simulink model "Aeropendulum"  (R2018b)
settings: Solver=VariableStepAuto  StartTime=0.0  StopTime=5  FixedStep=1e-3  MaxStep=1e-3  RelTol=1e-3
InitFcn:
  | mm = (0.008+0.0004+0.0034+2*0.0024);
  | mh = 0.007;
  | r = 0.012;
  | L = 0.285;
  | J = (mh*L^2)/3 + (2*mm*r^2)/5 + mm*(L+r)^2;
  | 
  | 
  | % where: mm = mass of the motor-propeller assembly
  | %            mh  = mass of the rod
  | 
  | coef = 0.0074;
  | 
  | A = -3.8099e-3;
  | B = 39.1002e-3;
  | C =  3.1245e-3;
  | D =  0;
  | 
  | fcpb = 2000;
libraries: simulink x1, vrlib x1, powerlib x1
settings Model: Creator=user  LastModifiedBy=user
settings CodeAppCC: StateflowObjectComments=on

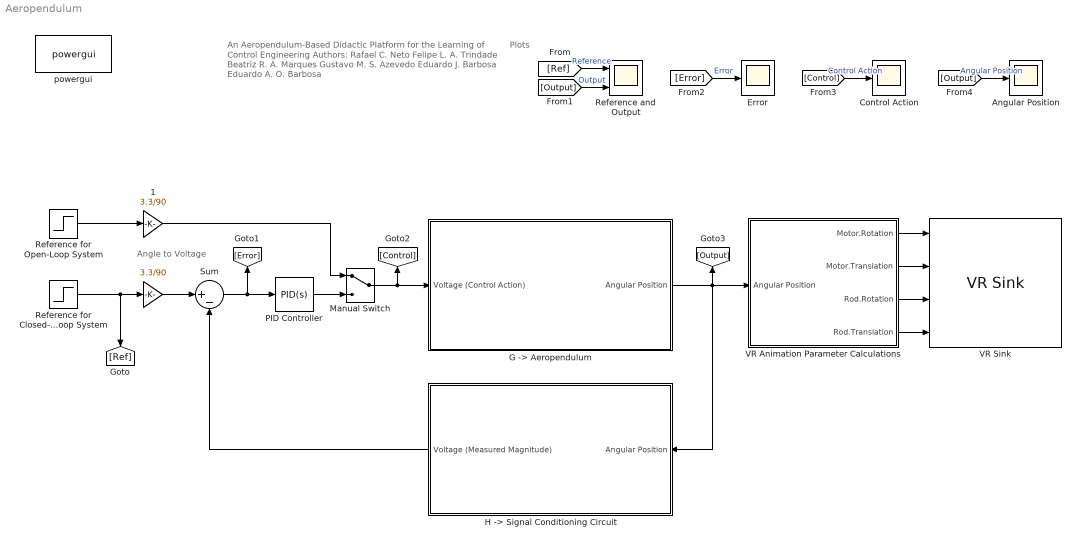
== system Aeropendulum ==
  note: Plots
  note: Angle to
      | Voltage
  note: An Aeropendulum-Based Didactic Platform
      | for the Learning of Control Engineering
      |
      | Authors: Rafael C. Neto
      | Felipe L. A. Trindade
      | Beatriz R. A. Marques
      | Gustavo M. S. Azevedo
      | Eduardo J. Barbosa
      | Eduardo A. O. Barbosa
  " " : Gain  Gain=3.3/90
  " 1" : Gain  Gain=3.3/90
  Angular Position : Scope
  Control Action : Scope
  Error : Scope
  "G -> Aeropendulum" : Subsystem  InitFcn=|
      | mm = (8+0.4+3.4+2*2.4)/1000  ; % motor + helice + parafusos + acrilico
      | mh = 0.007;
      | r = 0.03;
      | l = 0.25;
      | J = (mh*l^2/2) + (2*mm*r^2)/5 + mm*l^2;
  "H -> Signal Conditioning Circuit" : Subsystem
  Manual Switch : ManualSwitch
  PID Controller : simulink/Continuous/PID Controller  Controller=PID  Form=Parallel  TimeDomain=Continuous-time  SampleTime=-1  IntegratorMethod=Forward Euler  FilterMethod=Forward Euler  ControllerParametersSource=internal  P=0.095  I=0.95  D=0  UseFilter=on  N=100  TunerSelectOption=Transfer Function Based (PID Tuner App)  InitialConditionSource=internal  InitialConditionForIntegrator=0  InitialConditionForFilter=0  DifferentiatorICPrevScaledInput=0  ExternalReset=none  TrackingMode=off  Kt=1  LimitOutput=off  UpperSaturationLimit=inf  LowerSaturationLimit=-inf  LinearizeAsGain=on  AntiWindupMode=none  Kb=1  POutMin=[]  POutMax=[]  IOutMin=[]  IOutMax=[]  DOutMin=[]  DOutMax=[]  NOutMin=[]  NOutMax=[]  SumOutMin=[]  SumOutMax=[]  SaturationOutMin=[]  SaturationOutMax=[]  PParamMin=[]  PParamMax=[]  IParamMin=[]  IParamMax=[]  DParamMin=[]  DParamMax=[]  NParamMin=[]  NParamMax=[]  KbParamMin=[]  KbParamMax=[]  KtParamMin=[]  KtParamMax=[]  KbOutMin=[]  KbOutMax=[]  KtOutMin=[]  KtOutMax=[]  IntegratorOutMin=[]  IntegratorOutMax=[]  FilterOutMin=[]  FilterOutMax=[]  SumI1OutMin=[]  SumI1OutMax=[]  SumI2OutMin=[]  SumI2OutMax=[]  SumI3OutMin=[]  SumI3OutMax=[]  SumI4OutMin=[]  SumI4OutMax=[]  SumDOutMin=[]  SumDOutMax=[]  DifferentiatorOutMin=[]  DifferentiatorOutMax=[]  FilterDiffOutCoefMin=[]  FilterDiffOutCoefMax=[]  ReciprocalOutMin=[]  ReciprocalOutMax=[]  SumDenOutMin=[]  SumDenOutMax=[]  SumNumOutMin=[]  SumNumOutMax=[]  DivideOutMin=[]  DivideOutMax=[]  IntegratorContinuousStateAttributes=''  IntegratorStateMustResolveToSignalObject=off  IntegratorRTWStateStorageClass=Auto  FilterContinuousStateAttributes=''  FilterStateMustResolveToSignalObject=off  FilterRTWStateStorageClass=Auto  ParallelPVariant=InternalParameters  IdealPVariant=Disabled  IVariant=InternalParameters  DVariant=InternalParameters  IntegratorVariant=Continuous  SatVariant=Disabled  AWVariant=Passthrough  PCopyVariant=Disabled  TRVariant=Disabled  FdbkBlocksVariant=Forward  IdealPFdbkVariant=Disabled  SatFdbkVariant=Disabled  DerivativeFilterVariant=ContFilter  NVariant=InternalParameters  NCopyVariant=Disabled  FilterICVariant=InternalICsFilter  IntegratorICVariant=InternalICs  ExternalResetVariant=Disabled  TRSumVariant=Passthrough  SumFdbkVariant=Disabled  SumVariant=Sum_PID
  Reference and Output : Scope  NumInputPorts=2
  Reference for Closed-Loop System : Step  After=55  SampleTime=0
  Reference for Open-Loop System : Step  After=55  SampleTime=0
  Sum : Sum  Inputs=|+-
  VR Animation Parameter Calculations : Subsystem
  VR Sink : vrlib/VR Sink  InstantiateOnLoad=on  SampleTime=0.01  ViewEnable=on  RemoteChange=off  RemoteView=off  FieldsWritten=Motor.rotation.4.1.1.double#Motor.translation.3.1.1.double#Haste.rotation.4.1.1.double#Haste.translation.3.1.1.double  WorldFileName=VRML_Aeropendulum.WRL  AutoView=off  VideoDimensions=[]  AllowVariableSize=off
      settings: SourceProductName=Simulink
  powergui : powerlib/powergui  Priority=1  SimulationMode=Discrete  SampleTime=1e-3  frequency=60  Iterations=50  frequencyindice=0  Pbase=100e6  ErrMax=1e-4  UnitsV=kV  UnitsW=MW  buscounter=0  FunctionMessages=off  echomessages=off  EnableUseOfTLC=off  CurrentSourceSwitches=off  DisableSnubberDevices=off  DisableRonSwitches=off  DisableVfSwitches=off  DisplayEquations=off  SolverType=Tustin/Backward Euler (TBE)  Interpol=off  ExternalGateDelay=off  methode=off  Ts=100  x0status=blocks  SPID=off  SwTol=0  HookPort=off  RestoreLinks=warning  ResistiveCurrentMeasurement=off  Frange=[0:2:500]  Ylog=off  Xlog=on  ShowGrid=off  save=off  variable=ZData  structure=0  ZoomFFT=off  StartTime=0.0  cycles=1  DisplayStyle=1  fundamental=60  FreqAxis=off  MaxFrequency=1000  frequencyindicesteady=1  RmsSteady=1  display=off
  wires:
  "G -> Aeropendulum"/1(Angular Position) -> "H -> Signal Conditioning Circuit"/1(Angular Position), VR Animation Parameter Calculations/1(Angular Position), [Output]
  "H -> Signal Conditioning Circuit"/1(Voltage (Measured Magnitude)) -> Sum/2
  Reference for Closed-Loop System/1 -> " "/1, [Ref]
  Sum/1 -> PID Controller/1, [Error]
  VR Animation Parameter Calculations/1(Motor.Rotation) -> VR Sink/1
  VR Animation Parameter Calculations/2(Motor.Translation) -> VR Sink/2
  VR Animation Parameter Calculations/3(Rod.Rotation) -> VR Sink/3
  VR Animation Parameter Calculations/4(Rod.Translation) -> VR Sink/4
  Manual Switch/1 -> "G -> Aeropendulum"/1(Voltage (Control Action)), [Control]
  Reference for Open-Loop System/1 -> " 1"/1
  PID Controller/1 -> Manual Switch/2
  " "/1 -> Sum/1
  [Ref] -> Reference and Output/1  "Reference"
  [Output] -> Reference and Output/2  "Output"
  [Error] -> Error/1  "Error"
  [Control] -> Control Action/1  "Control Action"
  [Output] -> Angular Position/1  "Angular Position"
  " 1"/1 -> Manual Switch/1

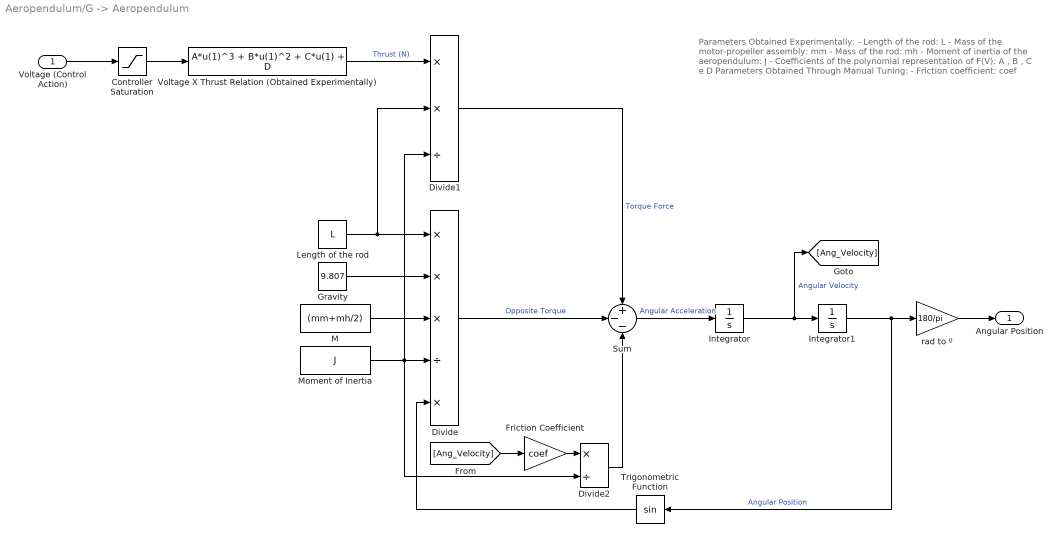
== system Aeropendulum/G -> Aeropendulum ==
  note: Parameters Obtained Experimentally:
      | - Length of the rod: L
      | - Mass of the motor-propeller assembly: mm
      | - Mass of the rod: mh
      | - Moment of inertia of the aeropendulum: J
      | - Coefficients of the polynomial
      | representation of F(V): A , B , C e D
      |
      | Parameters Obtained Through Manual Tuning:
      | - Friction coefficient: coef
  Voltage (Control Action) : Inport
  " Friction Coefficient" : Gain  Gain=coef
  Controller Saturation : Saturate  UpperLimit=3.7  LowerLimit=0
  Divide : Product  Inputs=***/*
  Divide1 : Product  Inputs=**/
  Divide2 : Product  Inputs=*/
  Gravity : Constant  Value=9.807
  Integrator : Integrator
  Integrator1 : Integrator
  Length of the rod : Constant  Value=L
  M : Constant  Value=(mm+mh/2)
  Moment of Inertia : Constant  Value=J
  Sum : Sum  Inputs=+--
  Trigonometric Function : Trigonometry
  Voltage X Thrust Relation (Obtained Experimentally) : Fcn  Expr=A*u(1)^3 + B*u(1)^2 + C*u(1) + D
  rad to º : Gain  Gain=180/pi
  Angular Position : Outport
  wires:
  Trigonometric Function/1 -> Divide/5
  Length of the rod/1 -> Divide1/2, Divide/1
  Moment of Inertia/1 -> Divide2/2, Divide1/3, Divide/4
  M/1 -> Divide/3
  Voltage (Control Action)/1 -> Controller Saturation/1
  Voltage X Thrust Relation (Obtained Experimentally)/1 -> Divide1/1  "Thrust (N)"
  Gravity/1 -> Divide/2
  Integrator/1 -> [Ang_Velocity], Integrator1/1  "Angular Velocity"
  Sum/1 -> Integrator/1  "Angular Acceleration"
  Integrator1/1 -> rad to º/1, Trigonometric Function/1  "Angular Position"
  Divide/1 -> Sum/2  "Opposite Torque"
  rad to º/1 -> Angular Position/1
  Divide1/1 -> Sum/1  "Torque Force"
  Controller Saturation/1 -> Voltage X Thrust Relation (Obtained Experimentally)/1
  [Ang_Velocity] -> " Friction Coefficient"/1
  " Friction Coefficient"/1 -> Divide2/1
  Divide2/1 -> Sum/3

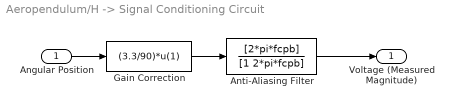
== system Aeropendulum/H -> Signal Conditioning Circuit ==
  Angular Position : Inport
  Anti-Aliasing Filter : TransferFcn  Numerator=[2*pi*fcpb]  Denominator=[1 2*pi*fcpb]
  Gain Correction : Fcn  Expr=(3.3/90)*u(1)
  Voltage (Measured Magnitude) : Outport
  wires:
  Gain Correction/1 -> Anti-Aliasing Filter/1
  Angular Position/1 -> Gain Correction/1
  Anti-Aliasing Filter/1 -> Voltage (Measured Magnitude)/1

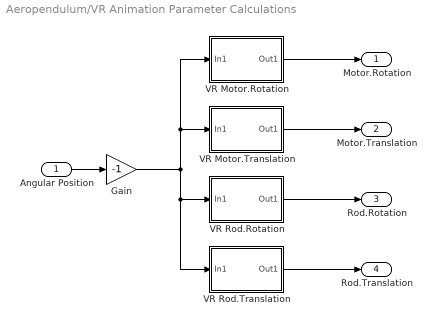
== system Aeropendulum/VR Animation Parameter Calculations ==
  Angular Position : Inport
  Gain : Gain  Gain=-1
  VR Motor.Rotation : Subsystem
  VR Motor.Translation : Subsystem
  VR Rod.Rotation : Subsystem
  VR Rod.Translation : Subsystem
  Motor.Rotation : Outport
  Motor.Translation : Outport  Port=2
  Rod.Rotation : Outport  Port=3
  Rod.Translation : Outport  Port=4
  wires:
  VR Rod.Translation/1(Out1) -> Rod.Translation/1
  Angular Position/1 -> Gain/1
  VR Rod.Rotation/1(Out1) -> Rod.Rotation/1
  VR Motor.Translation/1(Out1) -> Motor.Translation/1
  VR Motor.Rotation/1(Out1) -> Motor.Rotation/1
  Gain/1 -> VR Motor.Rotation/1(In1), VR Motor.Translation/1(In1), VR Rod.Translation/1(In1), VR Rod.Rotation/1(In1)

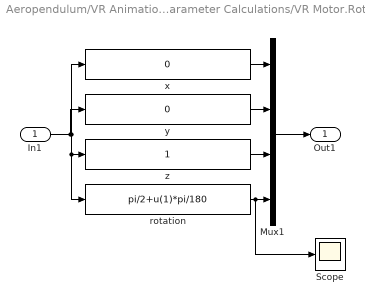
== system Aeropendulum/VR Animation Parameter Calculations/VR Motor.Rotation ==
  In1 : Inport
  Mux1 : Mux
  Scope : Scope
  rotation : Fcn  Expr=pi/2+u(1)*pi/180
  x : Fcn  Expr=0
  y : Fcn  Expr=0
  z : Fcn  Expr=1
  Out1 : Outport
  wires:
  Mux1/1 -> Out1/1
  In1/1 -> y/1, z/1, rotation/1, x/1
  y/1 -> Mux1/2
  x/1 -> Mux1/1
  rotation/1 -> Scope/1, Mux1/4
  z/1 -> Mux1/3

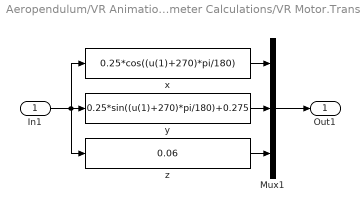
== system Aeropendulum/VR Animation Parameter Calculations/VR Motor.Translation ==
  In1 : Inport
  Mux1 : Mux  Inputs=3
  x : Fcn  Expr=0.25*cos((u(1)+270)*pi/180)
  y : Fcn  Expr=0.25*sin((u(1)+270)*pi/180)+0.275
  z : Fcn  Expr=0.06
  Out1 : Outport
  wires:
  x/1 -> Mux1/1
  y/1 -> Mux1/2
  In1/1 -> x/1, z/1, y/1
  z/1 -> Mux1/3
  Mux1/1 -> Out1/1

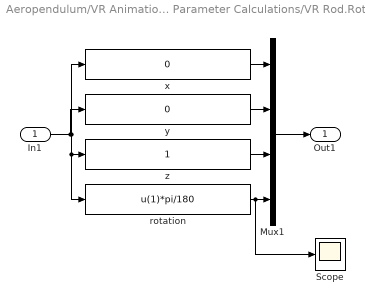
== system Aeropendulum/VR Animation Parameter Calculations/VR Rod.Rotation ==
  In1 : Inport
  Mux1 : Mux
  Scope : Scope
  rotation : Fcn  Expr=u(1)*pi/180
  x : Fcn  Expr=0
  y : Fcn  Expr=0
  z : Fcn  Expr=1
  Out1 : Outport
  wires:
  Mux1/1 -> Out1/1
  In1/1 -> y/1, z/1, rotation/1, x/1
  y/1 -> Mux1/2
  x/1 -> Mux1/1
  rotation/1 -> Scope/1, Mux1/4
  z/1 -> Mux1/3

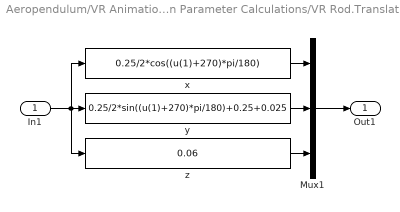
== system Aeropendulum/VR Animation Parameter Calculations/VR Rod.Translation ==
  In1 : Inport
  Mux1 : Mux  Inputs=3
  x : Fcn  Expr=0.25/2*cos((u(1)+270)*pi/180)
  y : Fcn  Expr=0.25/2*sin((u(1)+270)*pi/180)+0.25+0.025
  z : Fcn  Expr=0.06
  Out1 : Outport
  wires:
  x/1 -> Mux1/1
  y/1 -> Mux1/2
  In1/1 -> x/1, z/1, y/1
  z/1 -> Mux1/3
  Mux1/1 -> Out1/1
